simulink model "lab1"  (R2022b)
settings: Solver=VariableStepAuto  StartTime=0.0  StopTime=45  RelTol=1e-3
undefined symbols (not defined in the file or in its folder): degs2rpm, der, drv, gbox, mld, mot, pid, rads2rpm, rpm2rads, sens, Ts
libraries: simulink x3
settings Model: Creator=emanuelevitetta  LastModifiedBy=david

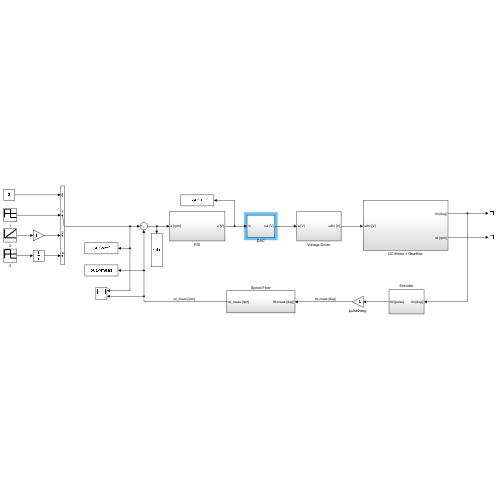
[thumbnail: Simulink's stored preview of the top-level diagram]
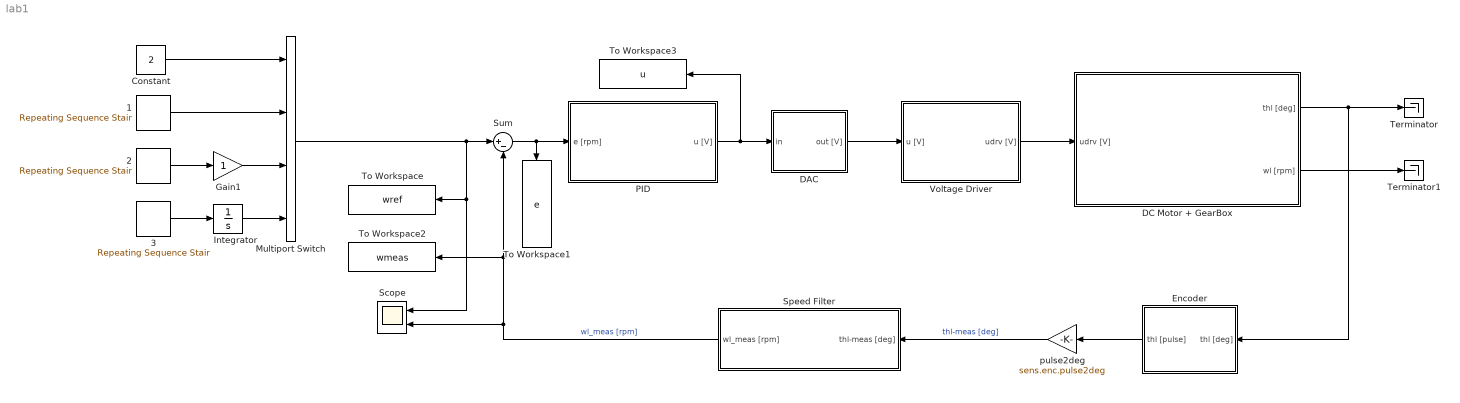
== system lab1 ==
  1 : simulink/Sources/Repeating Sequence Stair  OutValues=[250 -250].'  tsamp=1.5  OutMin=[]  OutMax=[]  OutDataTypeStr=double  OutputDataTypeScalingMode=double  OutDataType=fixdt(0,8)  ConRadixGroup=Best Precision: Vector-wise  OutScaling=2^-12
  2 : simulink/Sources/Repeating Sequence Stair  OutValues=[0 50 100 150 200 250 300 350 400 450 ].'  tsamp=5  OutMin=[]  OutMax=[]  OutDataTypeStr=double  OutputDataTypeScalingMode=double  OutDataType=fixdt(0,8)  ConRadixGroup=Best Precision: Vector-wise  OutScaling=2^-12
  3 : simulink/Sources/Repeating Sequence Stair  OutValues=[450 -450].'  tsamp=1  OutMin=[]  OutMax=[]  OutDataTypeStr=double  OutputDataTypeScalingMode=double  OutDataType=fixdt(0,8)  ConRadixGroup=Best Precision: Vector-wise  OutScaling=2^-12
  Constant : Constant  Value=2
  DAC : Subsystem
  DC Motor + GearBox : Subsystem
  Encoder : Subsystem
  Gain1 : Gain
  Integrator : Integrator
  Multiport Switch : MultiPortSwitch  SaturateOnIntegerOverflow=off  InputSameDT=off
  PID : Subsystem
  Scope : Scope  NumInputPorts=2
  Speed Filter : Subsystem
  Sum : Sum  Inputs=|+-
  Terminator : Terminator
  Terminator1 : Terminator
  To Workspace : ToWorkspace  VariableName=wref  SaveFormat=Timeseries  SampleTime=-1
  To Workspace1 : ToWorkspace  VariableName=e  SaveFormat=Timeseries  SampleTime=-1
  To Workspace2 : ToWorkspace  VariableName=wmeas  SaveFormat=Timeseries  SampleTime=-1
  To Workspace3 : ToWorkspace  VariableName=u  SaveFormat=Timeseries  SampleTime=-1
  Voltage Driver : Subsystem
  pulse2deg : Gain  Gain=sens.enc.pulse2deg
  wires:
  DC Motor + GearBox/1(thl [deg]) -> Encoder/1(thl [deg]), Terminator/1
  DC Motor + GearBox/2(wl [rpm]) -> Terminator1/1
  Voltage Driver/1(udrv [V]) -> DC Motor + GearBox/1(udrv [V])
  DAC/1(out [V]) -> Voltage Driver/1(u [V])
  PID/1(u [V]) -> To Workspace3/1, DAC/1(in)
  Encoder/1(thl [pulse]) -> pulse2deg/1
  Sum/1 -> To Workspace1/1, PID/1(e [rpm])
  pulse2deg/1 -> Speed Filter/1(thl-meas [deg])  "thl-meas [deg]"
  Speed Filter/1(wl_meas [rpm]) -> To Workspace2/1, Sum/2, Scope/2  "wl_meas [rpm]"
  Multiport Switch/1 -> Scope/1, To Workspace/1, Sum/1
  Gain1/1 -> Multiport Switch/3
  3/1 -> Integrator/1
  Constant/1 -> Multiport Switch/1
  1/1 -> Multiport Switch/2
  2/1 -> Gain1/1
  Integrator/1 -> Multiport Switch/4

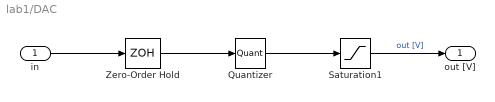
== system lab1/DAC ==
  in : Inport
  Quantizer : Quantizer  QuantizationInterval=daq.dac.q
  Saturation1 : Saturate  UpperLimit=10  LowerLimit=-10
  Zero-Order Hold : ZeroOrderHold  SampleTime=Ts
  out [V] : Outport
  wires:
  Saturation1/1 -> out [V]/1  "out [V]"
  in/1 -> Zero-Order Hold/1
  Zero-Order Hold/1 -> Quantizer/1
  Quantizer/1 -> Saturation1/1

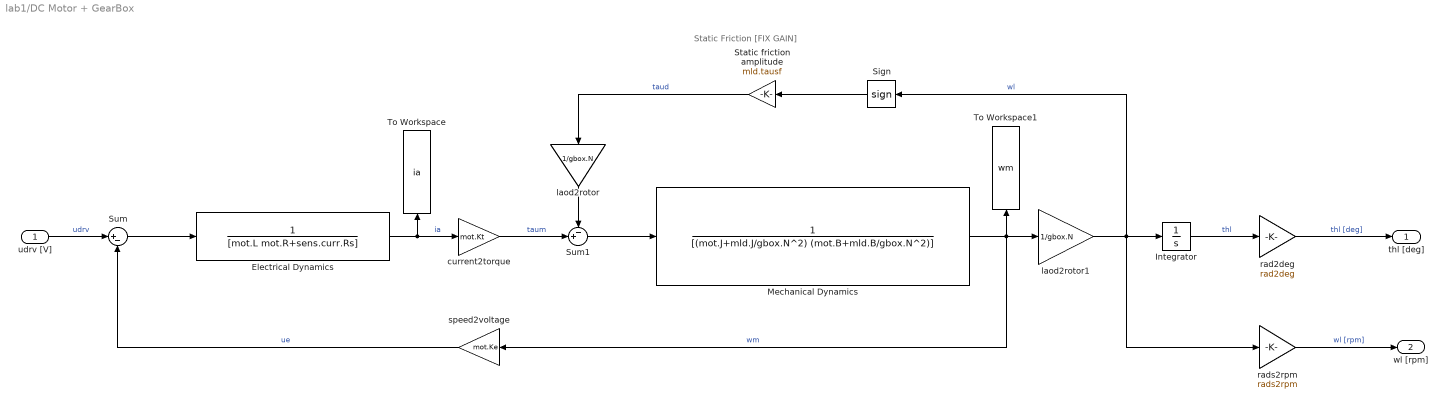
== system lab1/DC Motor + GearBox ==
  note: Static Friction [FIX GAIN]
  udrv [V] : Inport
  Electrical Dynamics : TransferFcn  Denominator=[mot.L mot.R+sens.curr.Rs]
  Integrator : Integrator
  Mechanical Dynamics : TransferFcn  Denominator=[(mot.J+mld.J/gbox.N^2) (mot.B+mld.B/gbox.N^2)]
  Sign : Signum  ZeroCross=off
  Static friction amplitude : Gain  Gain=mld.tausf
  Sum : Sum  Inputs=|+-
  Sum1 : Sum  Inputs=-+|
  To Workspace : ToWorkspace  VariableName=ia  SaveFormat=Timeseries  SampleTime=-1
  To Workspace1 : ToWorkspace  VariableName=wm  SaveFormat=Timeseries  SampleTime=-1
  current2torque : Gain  Gain=mot.Kt
  laod2rotor : Gain  Gain=1/gbox.N
  laod2rotor1 : Gain  Gain=1/gbox.N
  rad2deg : Gain  Gain=rad2deg
  rads2rpm : Gain  Gain=rads2rpm
  speed2voltage : Gain  Gain=mot.Ke
  thl [deg] : Outport
  wl [rpm] : Outport  Port=2
  wires:
  rads2rpm/1 -> wl [rpm]/1  "wl [rpm]"
  Sign/1 -> Static friction amplitude/1
  Electrical Dynamics/1 -> To Workspace/1, current2torque/1  "ia"
  Sum1/1 -> Mechanical Dynamics/1
  laod2rotor1/1 -> rads2rpm/1, Sign/1, Integrator/1  "wl"
  rad2deg/1 -> thl [deg]/1  "thl [deg]"
  laod2rotor/1 -> Sum1/1
  udrv [V]/1 -> Sum/1  "udrv"
  current2torque/1 -> Sum1/2  "taum"
  Static friction amplitude/1 -> laod2rotor/1  "taud"
  speed2voltage/1 -> Sum/2  "ue"
  Integrator/1 -> rad2deg/1  "thl"
  Sum/1 -> Electrical Dynamics/1
  Mechanical Dynamics/1 -> laod2rotor1/1, To Workspace1/1, speed2voltage/1  "wm"

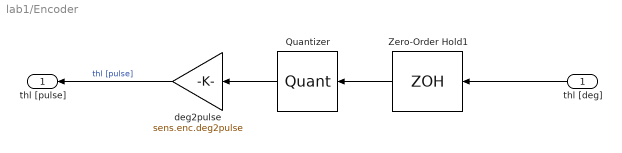
== system lab1/Encoder ==
  thl [deg] : Inport
  Quantizer : Quantizer  QuantizationInterval=sens.enc.pulse2deg
  Zero-Order Hold1 : ZeroOrderHold  SampleTime=Ts
  deg2pulse : Gain  Gain=sens.enc.deg2pulse
  thl [pulse] : Outport
  wires:
  thl [deg]/1 -> Zero-Order Hold1/1
  Zero-Order Hold1/1 -> Quantizer/1
  deg2pulse/1 -> thl [pulse]/1  "thl [pulse]"
  Quantizer/1 -> deg2pulse/1

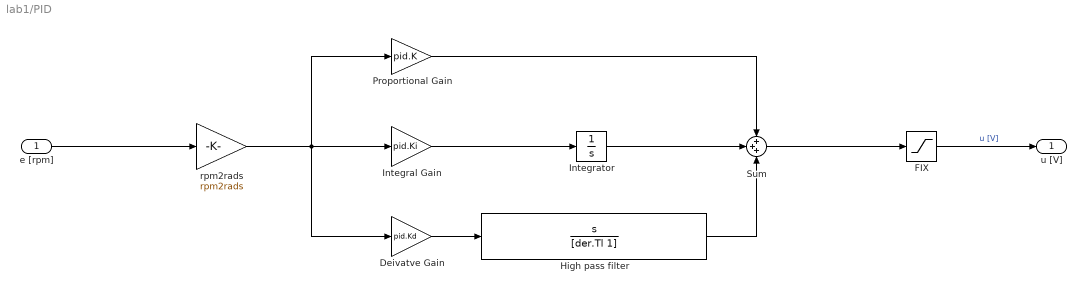
== system lab1/PID ==
  e [rpm] : Inport
  Deivatve Gain : Gain  Gain=pid.Kd
  "FIX " : Saturate  UpperLimit=10  LowerLimit=-10
  High pass filter : TransferFcn  Numerator=[1 0]  Denominator=[der.Tl 1]
  Integral Gain : Gain  Gain=pid.Ki
  Integrator : Integrator
  Proportional Gain : Gain  Gain=pid.K
  Sum : Sum  Inputs=+++
  rpm2rads : Gain  Gain=rpm2rads
  u [V] : Outport
  wires:
  Deivatve Gain/1 -> High pass filter/1
  e [rpm]/1 -> rpm2rads/1
  Integrator/1 -> Sum/2
  "FIX "/1 -> u [V]/1  "u [V]"
  rpm2rads/1 -> Deivatve Gain/1, Proportional Gain/1, Integral Gain/1
  High pass filter/1 -> Sum/3
  Integral Gain/1 -> Integrator/1
  Proportional Gain/1 -> Sum/1
  Sum/1 -> "FIX "/1

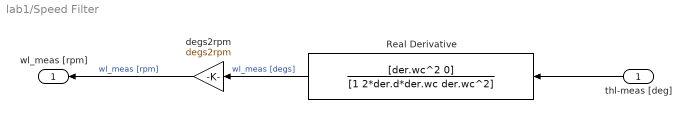
== system lab1/Speed Filter ==
  thl-meas [deg] : Inport
  Real Derivative : TransferFcn  Numerator=[der.wc^2 0]  Denominator=[1 2*der.d*der.wc der.wc^2]
  degs2rpm : Gain  Gain=degs2rpm
  wl_meas [rpm] : Outport
  wires:
  degs2rpm/1 -> wl_meas [rpm]/1  "wl_meas [rpm]"
  thl-meas [deg]/1 -> Real Derivative/1
  Real Derivative/1 -> degs2rpm/1  "wl_meas [degs]"

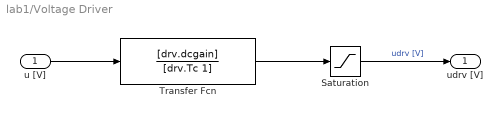
== system lab1/Voltage Driver ==
  u [V] : Inport
  Saturation : Saturate  UpperLimit=12  LowerLimit=-12
  Transfer Fcn : TransferFcn  Numerator=[drv.dcgain]  Denominator=[drv.Tc 1]
  udrv [V] : Outport
  wires:
  Saturation/1 -> udrv [V]/1  "udrv [V]"
  u [V]/1 -> Transfer Fcn/1
  Transfer Fcn/1 -> Saturation/1
